simulink library "functionAnglesSide"  (R2024a)
settings: Solver=VariableStepAuto  StartTime=0.0  StopTime=10.0  RelTol=1e-3
settings Model: Creator=renre  LastModifiedBy=renre

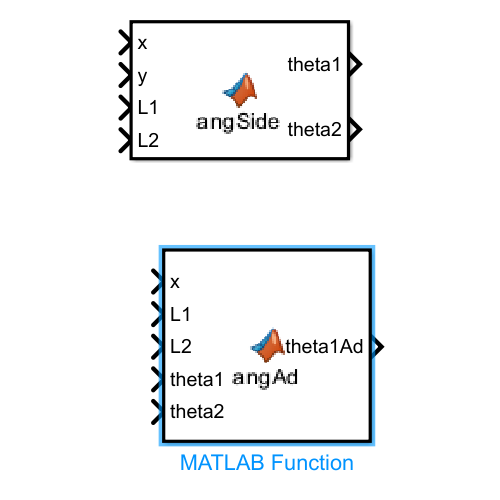
[thumbnail: Simulink's stored preview of the top-level diagram]
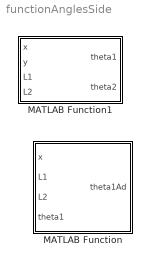
== system functionAnglesSide ==
  MATLAB Function : MATLAB Function  TreatAsAtomicUnit=on
  MATLAB Function1 : MATLAB Function  TreatAsAtomicUnit=on

== matlab function functionAnglesSide/MATLAB Function ==
  data: x input; theta1Ad output; L1 input; L2 input; theta1 input
function theta1Ad = angAd(x, L1, L2, theta1)

l = cos(theta1)*(L1 + L2);

theta1Ad = asin(-x/l);

== matlab function functionAnglesSide/MATLAB Function1 ==
  data: x input; theta1 output; y input; L1 input; L2 input; theta2 output
function [theta1, theta2] = angSide(x,y,L1,L2)
theta1 = atan(-x/y);
if theta1 ~= 0
    d = x / (2*sin(theta1));
    theta2 = acos(d/L1);
else
    d = -y/2;
    theta2 = acos(d/L1);
end
end
